simulink model "simulation_sine"  (R2023b)
settings: Solver=VariableStepAuto  StartTime=0.0  StopTime=t_end  RelTol=1e-3
InitFcn:
  | param = plant_param();
values from neighbouring files (symbols this model uses):
  Ts = (2*pi)/(100*w)    [plot_bode.m]
  w = w_vec(i)    [plot_bode.m]
settings Model: Creator=block  LastModifiedBy=block

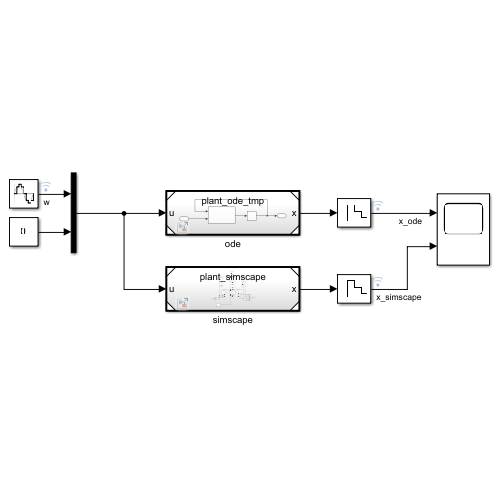
[thumbnail: Simulink's stored preview of the top-level diagram]
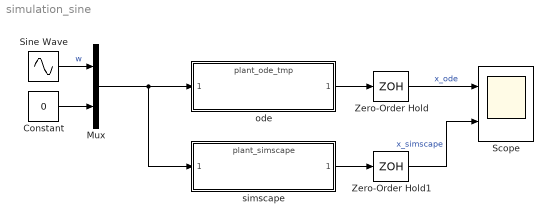
== system simulation_sine ==
  Constant : Constant  Value=0
  Mux : Mux  Inputs=2
  Scope : Scope  NumInputPorts=2
  Sine Wave : Sin  Frequency=w  SampleTime=Ts
  Zero-Order Hold : ZeroOrderHold  SampleTime=Ts
  Zero-Order Hold1 : ZeroOrderHold  SampleTime=Ts
  ode : ModelReference  ModelNameDialog=plant_ode_tmp  SimulationMode=Normal  ModelReferenceVersion=1.2
  simscape : ModelReference  ModelNameDialog=plant_simscape  SimulationMode=Normal  ModelReferenceVersion=1.8
  wires:
  Zero-Order Hold/1 -> Scope/1  "x_ode"
  simscape/1 -> Zero-Order Hold1/1
  Mux/1 -> simscape/1, ode/1
  ode/1 -> Zero-Order Hold/1
  Zero-Order Hold1/1 -> Scope/2  "x_simscape"
  Constant/1 -> Mux/2
  Sine Wave/1 -> Mux/1  "w"
